simulink model "InertialSimscape"  (R2017a)
settings: Solver=VariableStepAuto  StartTime=0.0  StopTime=10.0  RelTol=1e-3
values from neighbouring files (symbols this model uses):
  d1 = 0.2    [InertialMatlab.m]
  d2 = 1.0    (= 1)    [InertialMatlab.m]
  J1 = 0.4    [InertialMatlab.m]
  J2 = 1.0    (= 1)    [InertialMatlab.m]
libraries: fl_lib x10, nesl_utility x2
settings Model: Creator=mortenmj  LastModifiedBy=mortenmj

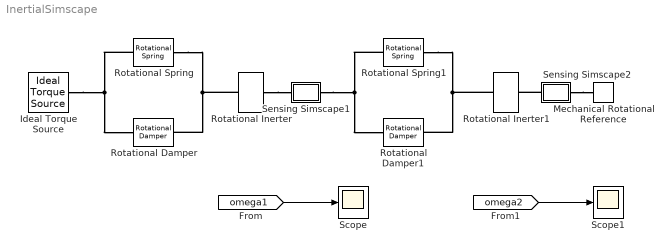
== system InertialSimscape ==
  Ideal Torque Source : fl_lib/Mechanical/Mechanical Sources/Ideal Torque Source
  Mechanical Rotational Reference : fl_lib/Mechanical/Rotational Elements/Mechanical Rotational Reference
  Rotational Damper : fl_lib/Mechanical/Rotational Elements/Rotational Damper  D=d1 N*m/(rad/s)  w_specify=off  w_priority=None  w=0 rad/s  w_nominal_specify=off  w_nominal_unit=rad/s  w_nominal_value=1  t_specify=off  t_priority=None  t=0 N*m  t_nominal_specify=off  t_nominal_unit=N*m  t_nominal_value=1
  Rotational Damper1 : fl_lib/Mechanical/Rotational Elements/Rotational Damper  D=d2 N*m/(rad/s)  w_specify=off  w_priority=None  w=0 rad/s  w_nominal_specify=off  w_nominal_unit=rad/s  w_nominal_value=1  t_specify=off  t_priority=None  t=0 N*m  t_nominal_specify=off  t_nominal_unit=N*m  t_nominal_value=1
  Rotational Inerter : fl_lib/Mechanical/Rotational Elements/Rotational Inerter  B=J1 kg*m^2  w_specify=off  w_priority=High  w=0 rad/s  w_nominal_specify=off  w_nominal_unit=rad/s  w_nominal_value=1  t_specify=off  t_priority=None  t=0 N*m  t_nominal_specify=off  t_nominal_unit=N*m  t_nominal_value=1
      settings: SourceProductName=Simscape  SourceProductBaseCode=SS
  Rotational Inerter1 : fl_lib/Mechanical/Rotational Elements/Rotational Inerter  B=J2 kg*m^2  w_specify=on  w_priority=High  w=1 rad/s  w_nominal_specify=off  w_nominal_unit=rad/s  w_nominal_value=1  t_specify=off  t_priority=None  t=0 N*m  t_nominal_specify=off  t_nominal_unit=N*m  t_nominal_value=1
      settings: SourceProductName=Simscape  SourceProductBaseCode=SS
  Rotational Spring : fl_lib/Mechanical/Rotational Elements/Rotational Spring  spr_rate=c1 N*m/rad  w_specify=off  w_priority=None  w=0 rad/s  w_nominal_specify=off  w_nominal_unit=rad/s  w_nominal_value=1  t_specify=off  t_priority=None  t=0 N*m  t_nominal_specify=off  t_nominal_unit=N*m  t_nominal_value=1  phi_specify=off  phi_priority=High  phi=0 rad  phi_nominal_specify=off  phi_nominal_unit=rad  phi_nominal_value=1
      settings: SourceProductName=Simscape
  Rotational Spring1 : fl_lib/Mechanical/Rotational Elements/Rotational Spring  spr_rate=c2 N*m/rad  w_specify=off  w_priority=None  w=0 rad/s  w_nominal_specify=off  w_nominal_unit=rad/s  w_nominal_value=1  t_specify=off  t_priority=None  t=0 N*m  t_nominal_specify=off  t_nominal_unit=N*m  t_nominal_value=1  phi_specify=off  phi_priority=High  phi=0 rad  phi_nominal_specify=off  phi_nominal_unit=rad  phi_nominal_value=1
      settings: SourceProductName=Simscape
  Scope : Scope
  Scope1 : Scope
  Sensing Simscape1 : Subsystem
      mask Display: disp('ω')
  Sensing Simscape2 : Subsystem
      mask Display: disp('ω')
  wires:
  [omega1] -> Scope/1
  [omega2] -> Scope1/1
  connections:
  Rotational Spring/LConn1 -- Ideal Torque Source/LConn1 -- Rotational Damper/LConn1
  Rotational Spring/RConn1 -- Rotational Inerter/LConn1 -- Rotational Damper/RConn1
  Rotational Spring1/RConn1 -- Rotational Inerter1/LConn1 -- Rotational Damper1/RConn1
  Rotational Spring1/LConn1 -- Sensing Simscape1/LConn1 -- Rotational Damper1/LConn1
  Sensing Simscape2/RConn1 -- Rotational Inerter1/RConn1
  Sensing Simscape2/LConn1 -- Mechanical Rotational Reference/LConn1
  Rotational Inerter/RConn1 -- Sensing Simscape1/RConn1

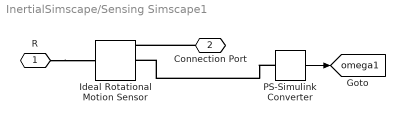
== system InertialSimscape/Sensing Simscape1 ==
  Ideal Rotational Motion Sensor : fl_lib/Mechanical/Mechanical Sensors/Ideal Rotational Motion Sensor  offset=0 rad
  PS-Simulink Converter : nesl_utility/PS-Simulink Converter  PhysicalDomain=network_engine_domain  SubClassName=ps_output  LeftPortType=input  RightPortType=output  PseudoPeriodic=off  Frequencies=[]  Unit=rad/s  AffineConversion=off
  R : PMIOPort  Port=1  Side=Left
  Connection Port : PMIOPort  Port=2  Side=Right
  tag scope: omega1=global
  wires:
  PS-Simulink Converter/1 -> [omega1]
  connections:
  R/RConn1 -- Ideal Rotational Motion Sensor/LConn1
  Connection Port/RConn1 -- Ideal Rotational Motion Sensor/RConn1
  PS-Simulink Converter/LConn1 -- Ideal Rotational Motion Sensor/RConn2

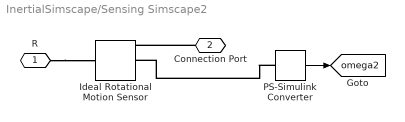
== system InertialSimscape/Sensing Simscape2 ==
  Ideal Rotational Motion Sensor : fl_lib/Mechanical/Mechanical Sensors/Ideal Rotational Motion Sensor  offset=0 rad
  PS-Simulink Converter : nesl_utility/PS-Simulink Converter  PhysicalDomain=network_engine_domain  SubClassName=ps_output  LeftPortType=input  RightPortType=output  PseudoPeriodic=off  Frequencies=[]  Unit=rad/s  AffineConversion=off
  R : PMIOPort  Port=1  Side=Left
  Connection Port : PMIOPort  Port=2  Side=Right
  tag scope: omega2=global
  wires:
  PS-Simulink Converter/1 -> [omega2]
  connections:
  R/RConn1 -- Ideal Rotational Motion Sensor/LConn1
  Connection Port/RConn1 -- Ideal Rotational Motion Sensor/RConn1
  PS-Simulink Converter/LConn1 -- Ideal Rotational Motion Sensor/RConn2
